simulink model "uavModelModifiedOld"  (R2019a)
settings: Solver=VariableStepAuto  StartTime=0.0  StopTime=50  RelTol=1e-3
undefined symbols (not defined in the file or in its folder): Motor
libraries: simulink x8
(part 1 of 2)
settings Model: Creator=tdarrah  LastModifiedBy=tdarrah
settings DataIOCC: ReturnWorkspaceOutputs=off
settings DebuggingCC: ArithmeticOperatorsInVariantConditions=warning
settings SFSimCC: SimUseLocalCustomCode=off
settings RTWCC: RTWUseLocalCustomCode=off
settings CodeAppCC: StateflowObjectComments=on

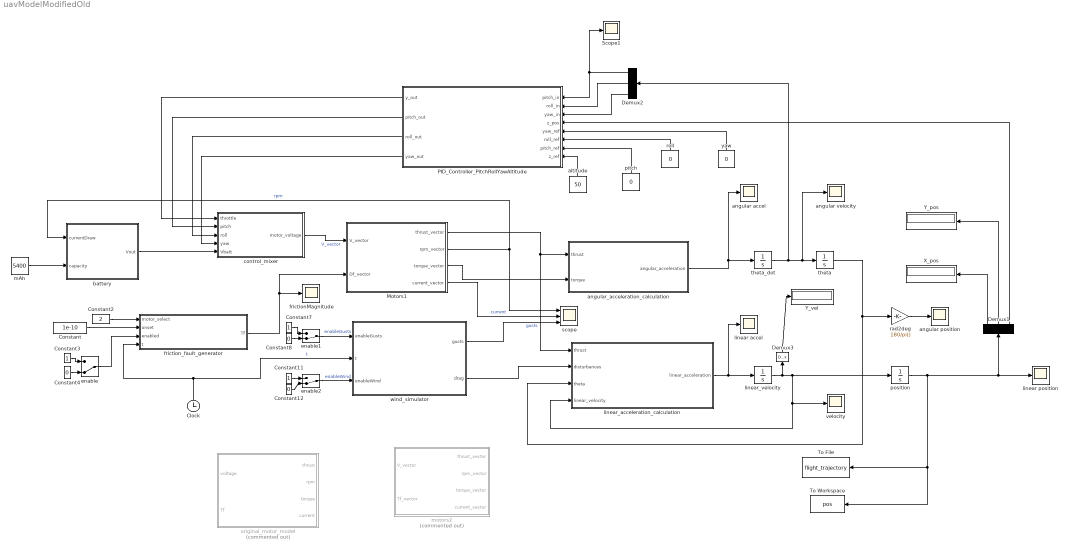
== system uavModelModifiedOld ==
  Clock : Clock
  Constant : Constant  Value=1e-10
  Constant11 : Constant
  Constant12 : Constant  Value=0
  Constant2 : Constant  Value=2
  Constant3 : Constant
  Constant4 : Constant  Value=0
  Constant7 : Constant
  Constant8 : Constant  Value=0
  Demux1 : Demux  Outputs=3
  Demux2 : Demux  Outputs=3
  Demux3 : Demux  Outputs=3
  Motors1 : Subsystem
  PID_Controller_PitchRollYawAltitude : Subsystem
  Scope1 : Scope
  To File : ToFile  Filename=flight_trajectory  MatrixName=pos  SampleTime=.1
  To Workspace : ToWorkspace  VariableName=pos  SampleTime=-1
      settings: Save2DSignal=2-D array (concatenate along first dimension)
  X_pos : Display
  Y_pos : Display
  Y_vel : Display
  altitude : Constant  Value=50
  angular accel : Scope
  angular position : Scope
  angular velocity : Scope
  angular_acceleration_calculation : MATLAB Function  TreatAsAtomicUnit=on
  battery : Subsystem
  control_mixer : MATLAB Function  TreatAsAtomicUnit=on
  enable : ManualSwitch  CurrentSetting=0
  enable1 : ManualSwitch  CurrentSetting=0
  enable2 : ManualSwitch  CurrentSetting=0
  frictionMagnitude : Scope
  friction_fault_generator : MATLAB Function  TreatAsAtomicUnit=on
  linear accel : Scope
  linear position : Scope
  linear_acceleration_calculation : MATLAB Function  TreatAsAtomicUnit=on
  linear_velocity : Integrator
  mAh : Constant  Value=5400
  motors2 : Subsystem  Commented=on
  original_motor_model : MATLAB Function  Commented=on  TreatAsAtomicUnit=on
  pitch : Constant  Value=0
  "position " : Integrator
  rad2deg : Gain  Gain=180/pi()
  roll : Constant  Value=0
  scope : Scope  NumInputPorts=3
  theta : Integrator
  theta_dot : Integrator
  velocity : Scope
  wind_simulator : Subsystem
  yaw : Constant  Value=0
  wires:
  Motors1/1(thrust_vector) -> linear_acceleration_calculation/1(thrust), angular_acceleration_calculation/1(thrust)
  Motors1/3(torque_vector) -> angular_acceleration_calculation/2(torque)
  angular_acceleration_calculation/1(angular_acceleration) -> angular accel/1, theta_dot/1
  theta_dot/1 -> Demux2/1, angular velocity/1, theta/1
  linear_acceleration_calculation/1(linear_acceleration) -> linear accel/1, linear_velocity/1
  linear_velocity/1 -> "position "/1, linear_acceleration_calculation/4(linear_velocity), velocity/1, Demux3/1
  rad2deg/1 -> angular position/1
  theta/1 -> rad2deg/1, linear_acceleration_calculation/3(theta)
  control_mixer/1(motor_voltage) -> Motors1/1(V_vector)  "V_vector"
  Motors1/4(current_vector) -> scope/2  "current"
  battery/1(Vout) -> control_mixer/5(Vbatt)
  Demux2/1 -> PID_Controller_PitchRollYawAltitude/1(pitch_in), Scope1/1
  Demux2/2 -> PID_Controller_PitchRollYawAltitude/2(roll_in)
  Demux2/3 -> PID_Controller_PitchRollYawAltitude/3(yaw_in)
  Demux1/3 -> PID_Controller_PitchRollYawAltitude/4(z_pos)
  PID_Controller_PitchRollYawAltitude/1(y_out) -> control_mixer/1(throttle)
  PID_Controller_PitchRollYawAltitude/2(pitch_out) -> control_mixer/2(pitch)
  PID_Controller_PitchRollYawAltitude/3(roll_out) -> control_mixer/3(roll)
  PID_Controller_PitchRollYawAltitude/4(yaw_out) -> control_mixer/4(yaw)
  altitude/1 -> PID_Controller_PitchRollYawAltitude/8(z_ref)
  roll/1 -> PID_Controller_PitchRollYawAltitude/6(roll_ref)
  yaw/1 -> PID_Controller_PitchRollYawAltitude/5(yaw_ref)
  Clock/1 -> wind_simulator/2(t), friction_fault_generator/4(t)  "t"
  friction_fault_generator/1(Tf) -> frictionMagnitude/1, Motors1/2(Df_vector)
  Constant2/1 -> friction_fault_generator/1(motor_select)
  Constant3/1 -> enable/1
  enable/1 -> friction_fault_generator/3(enabled)
  Constant4/1 -> enable/2
  Motors1/2(rpm_vector) -> battery/1(currentDraw), scope/1  "rpm"
  "position "/1 -> linear position/1, Demux1/1, To File/1, To Workspace/1
  Constant/1 -> friction_fault_generator/2(onset)
  mAh/1 -> battery/2(capacity)
  wind_simulator/1(gusts) -> scope/3  "gusts"
  wind_simulator/2(drag) -> linear_acceleration_calculation/2(disturbances)
  Demux1/1 -> X_pos/1
  Demux1/2 -> Y_pos/1
  Constant7/1 -> enable1/1
  Constant8/1 -> enable1/2
  enable1/1 -> wind_simulator/1(enableGusts)  "enableGusts"
  Constant11/1 -> enable2/1
  enable2/1 -> wind_simulator/3(enableWind)  "enableWind"
  Constant12/1 -> enable2/2
  Demux3/2 -> Y_vel/1
  pitch/1 -> PID_Controller_PitchRollYawAltitude/7(pitch_ref)

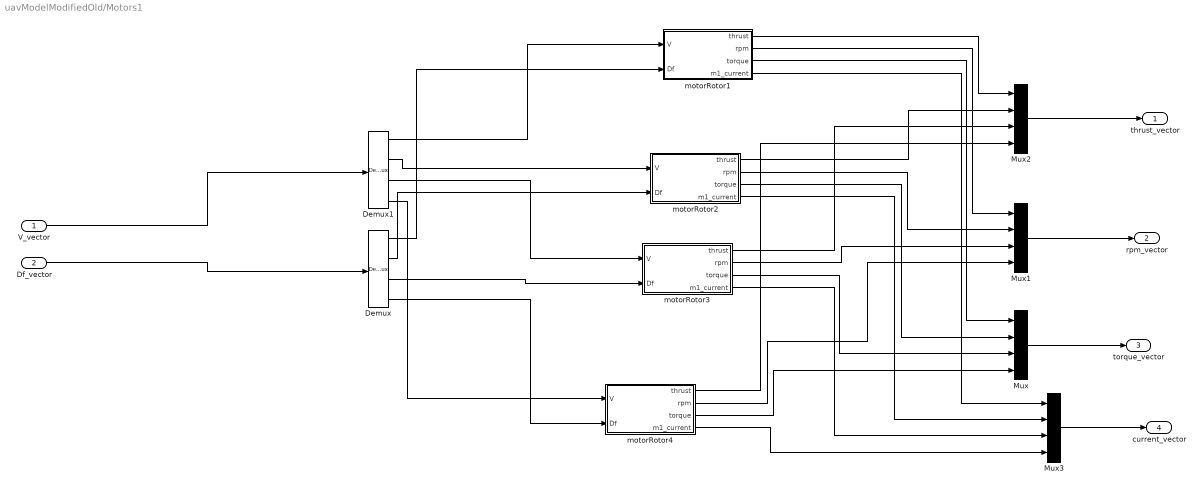
== system uavModelModifiedOld/Motors1 ==
  V_vector : Inport
  Df_vector : Inport  Port=2
  Demux : Demux
  Demux1 : Demux
  Mux{,1..3} (4 alike) : Mux
  motorRotor1 : Subsystem
  motorRotor2 : Subsystem
  motorRotor3 : Subsystem
  motorRotor4 : Subsystem
  thrust_vector : Outport
  rpm_vector : Outport  Port=2
  torque_vector : Outport  Port=3
  current_vector : Outport  Port=4
  wires:
  motorRotor4/3(torque) -> Mux/4
  motorRotor1/2(rpm) -> Mux1/1
  Mux1/1 -> rpm_vector/1
  Demux1/3 -> motorRotor3/1(V)
  V_vector/1 -> Demux1/1
  motorRotor1/1(thrust) -> Mux2/1
  motorRotor4/1(thrust) -> Mux2/4
  motorRotor3/2(rpm) -> Mux1/3
  motorRotor2/2(rpm) -> Mux1/2
  motorRotor2/3(torque) -> Mux/2
  Mux2/1 -> thrust_vector/1
  motorRotor1/3(torque) -> Mux/1
  motorRotor3/3(torque) -> Mux/3
  motorRotor4/2(rpm) -> Mux1/4
  motorRotor2/1(thrust) -> Mux2/2
  motorRotor3/1(thrust) -> Mux2/3
  Demux1/1 -> motorRotor1/1(V)
  Demux/2 -> motorRotor2/2(Df)
  Demux/3 -> motorRotor3/2(Df)
  Demux/1 -> motorRotor1/2(Df)
  Df_vector/1 -> Demux/1
  Demux1/4 -> motorRotor4/1(V)
  Mux/1 -> torque_vector/1
  Demux1/2 -> motorRotor2/1(V)
  Demux/4 -> motorRotor4/2(Df)
  motorRotor1/4(m1_current) -> Mux3/1
  Mux3/1 -> current_vector/1
  motorRotor2/4(m1_current) -> Mux3/2
  motorRotor3/4(m1_current) -> Mux3/3
  motorRotor4/4(m1_current) -> Mux3/4

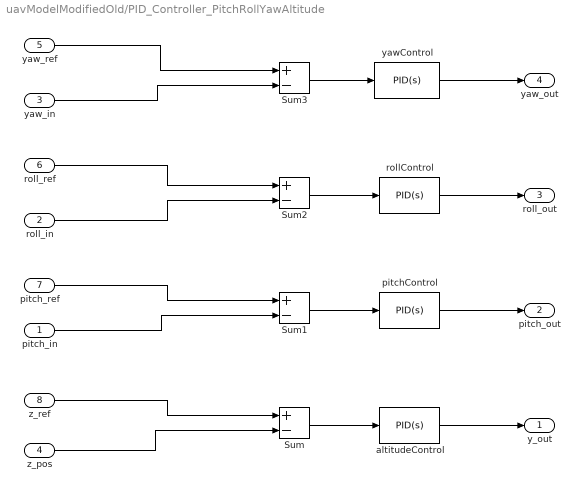
== system uavModelModifiedOld/PID_Controller_PitchRollYawAltitude ==
  pitch_in : Inport
  roll_in : Inport  Port=2
  yaw_in : Inport  Port=3
  z_pos : Inport  Port=4
  yaw_ref : Inport  Port=5
  roll_ref : Inport  Port=6
  pitch_ref : Inport  Port=7
  z_ref : Inport  Port=8
  Sum{,1..3} (4 alike) : Sum  Inputs=+-
  altitudeControl : simulink/Continuous/PID Controller  Controller=PID  Form=Parallel  TimeDomain=Continuous-time  SampleTime=-1  IntegratorMethod=Forward Euler  FilterMethod=Forward Euler  ControllerParametersSource=internal  P=9.031  I=1  D=10  UseFilter=on  N=100  TunerSelectOption=Transfer Function Based (PID Tuner App)  InitialConditionSource=internal  InitialConditionForIntegrator=0  InitialConditionForFilter=0  DifferentiatorICPrevScaledInput=0  ExternalReset=none  TrackingMode=off  Kt=1  LimitOutput=on  UpperSaturationLimit=100  LowerSaturationLimit=0  LinearizeAsGain=on  AntiWindupMode=clamping  Kb=1  POutMin=[]  POutMax=[]  IOutMin=[]  IOutMax=[]  DOutMin=[]  DOutMax=[]  NOutMin=[]  NOutMax=[]  SumOutMin=[]  SumOutMax=[]  SaturationOutMin=[]  SaturationOutMax=[]  PParamMin=[]  PParamMax=[]  IParamMin=[]  IParamMax=[]  DParamMin=[]  DParamMax=[]  NParamMin=[]  NParamMax=[]  KbParamMin=[]  KbParamMax=[]  KtParamMin=[]  KtParamMax=[]  KbOutMin=[]  KbOutMax=[]  KtOutMin=[]  KtOutMax=[]  IntegratorOutMin=[]  IntegratorOutMax=[]  FilterOutMin=[]  FilterOutMax=[]  SumI1OutMin=[]  SumI1OutMax=[]  SumI2OutMin=[]  SumI2OutMax=[]  SumI3OutMin=[]  SumI3OutMax=[]  SumI4OutMin=[]  SumI4OutMax=[]  SumDOutMin=[]  SumDOutMax=[]  DifferentiatorOutMin=[]  DifferentiatorOutMax=[]  FilterDiffOutCoefMin=[]  FilterDiffOutCoefMax=[]  ReciprocalOutMin=[]  ReciprocalOutMax=[]  SumDenOutMin=[]  SumDenOutMax=[]  SumNumOutMin=[]  SumNumOutMax=[]  DivideOutMin=[]  DivideOutMax=[]  IntegratorContinuousStateAttributes=''  IntegratorStateMustResolveToSignalObject=off  IntegratorRTWStateStorageClass=Auto  FilterContinuousStateAttributes=''  FilterStateMustResolveToSignalObject=off  FilterRTWStateStorageClass=Auto  ParallelPVariant=InternalParameters  IdealPVariant=Disabled  IVariant=InternalParameters  DVariant=InternalParameters  IntegratorVariant=Continuous  SatVariant=Enabled  AWVariant=ContClampingParallel  PCopyVariant=Disabled  TRVariant=Disabled  FdbkBlocksVariant=Forward  IdealPFdbkVariant=Disabled  SatFdbkVariant=Disabled  DerivativeFilterVariant=ContFilter  NVariant=InternalParameters  NCopyVariant=Disabled  FilterICVariant=InternalICsFilter  IntegratorICVariant=InternalICs  ExternalResetVariant=Disabled  TRSumVariant=Passthrough  SumFdbkVariant=Disabled  SumVariant=Sum_PID
  pitchControl : simulink/Continuous/PID Controller  Controller=PID  Form=Parallel  TimeDomain=Continuous-time  SampleTime=-1  IntegratorMethod=Forward Euler  FilterMethod=Forward Euler  ControllerParametersSource=internal  P=15  I=5  D=0  UseFilter=on  N=100  TunerSelectOption=Transfer Function Based (PID Tuner App)  InitialConditionSource=internal  InitialConditionForIntegrator=0  InitialConditionForFilter=0  DifferentiatorICPrevScaledInput=0  ExternalReset=none  TrackingMode=off  Kt=1  LimitOutput=on  UpperSaturationLimit=100  LowerSaturationLimit=0  LinearizeAsGain=on  AntiWindupMode=clamping  Kb=1  POutMin=[]  POutMax=[]  IOutMin=[]  IOutMax=[]  DOutMin=[]  DOutMax=[]  NOutMin=[]  NOutMax=[]  SumOutMin=[]  SumOutMax=[]  SaturationOutMin=[]  SaturationOutMax=[]  PParamMin=[]  PParamMax=[]  IParamMin=[]  IParamMax=[]  DParamMin=[]  DParamMax=[]  NParamMin=[]  NParamMax=[]  KbParamMin=[]  KbParamMax=[]  KtParamMin=[]  KtParamMax=[]  KbOutMin=[]  KbOutMax=[]  KtOutMin=[]  KtOutMax=[]  IntegratorOutMin=[]  IntegratorOutMax=[]  FilterOutMin=[]  FilterOutMax=[]  SumI1OutMin=[]  SumI1OutMax=[]  SumI2OutMin=[]  SumI2OutMax=[]  SumI3OutMin=[]  SumI3OutMax=[]  SumI4OutMin=[]  SumI4OutMax=[]  SumDOutMin=[]  SumDOutMax=[]  DifferentiatorOutMin=[]  DifferentiatorOutMax=[]  FilterDiffOutCoefMin=[]  FilterDiffOutCoefMax=[]  ReciprocalOutMin=[]  ReciprocalOutMax=[]  SumDenOutMin=[]  SumDenOutMax=[]  SumNumOutMin=[]  SumNumOutMax=[]  DivideOutMin=[]  DivideOutMax=[]  IntegratorContinuousStateAttributes=''  IntegratorStateMustResolveToSignalObject=off  IntegratorRTWStateStorageClass=Auto  FilterContinuousStateAttributes=''  FilterStateMustResolveToSignalObject=off  FilterRTWStateStorageClass=Auto  ParallelPVariant=InternalParameters  IdealPVariant=Disabled  IVariant=InternalParameters  DVariant=InternalParameters  IntegratorVariant=Continuous  SatVariant=Enabled  AWVariant=ContClampingParallel  PCopyVariant=Disabled  TRVariant=Disabled  FdbkBlocksVariant=Forward  IdealPFdbkVariant=Disabled  SatFdbkVariant=Disabled  DerivativeFilterVariant=ContFilter  NVariant=InternalParameters  NCopyVariant=Disabled  FilterICVariant=InternalICsFilter  IntegratorICVariant=InternalICs  ExternalResetVariant=Disabled  TRSumVariant=Passthrough  SumFdbkVariant=Disabled  SumVariant=Sum_PID
  rollControl : simulink/Continuous/PID Controller  Controller=PID  Form=Parallel  TimeDomain=Continuous-time  SampleTime=-1  IntegratorMethod=Forward Euler  FilterMethod=Forward Euler  ControllerParametersSource=internal  P=15  I=5  D=0  UseFilter=on  N=100  TunerSelectOption=Transfer Function Based (PID Tuner App)  InitialConditionSource=internal  InitialConditionForIntegrator=0  InitialConditionForFilter=0  DifferentiatorICPrevScaledInput=0  ExternalReset=none  TrackingMode=off  Kt=1  LimitOutput=on  UpperSaturationLimit=100  LowerSaturationLimit=0  LinearizeAsGain=on  AntiWindupMode=clamping  Kb=1  POutMin=[]  POutMax=[]  IOutMin=[]  IOutMax=[]  DOutMin=[]  DOutMax=[]  NOutMin=[]  NOutMax=[]  SumOutMin=[]  SumOutMax=[]  SaturationOutMin=[]  SaturationOutMax=[]  PParamMin=[]  PParamMax=[]  IParamMin=[]  IParamMax=[]  DParamMin=[]  DParamMax=[]  NParamMin=[]  NParamMax=[]  KbParamMin=[]  KbParamMax=[]  KtParamMin=[]  KtParamMax=[]  KbOutMin=[]  KbOutMax=[]  KtOutMin=[]  KtOutMax=[]  IntegratorOutMin=[]  IntegratorOutMax=[]  FilterOutMin=[]  FilterOutMax=[]  SumI1OutMin=[]  SumI1OutMax=[]  SumI2OutMin=[]  SumI2OutMax=[]  SumI3OutMin=[]  SumI3OutMax=[]  SumI4OutMin=[]  SumI4OutMax=[]  SumDOutMin=[]  SumDOutMax=[]  DifferentiatorOutMin=[]  DifferentiatorOutMax=[]  FilterDiffOutCoefMin=[]  FilterDiffOutCoefMax=[]  ReciprocalOutMin=[]  ReciprocalOutMax=[]  SumDenOutMin=[]  SumDenOutMax=[]  SumNumOutMin=[]  SumNumOutMax=[]  DivideOutMin=[]  DivideOutMax=[]  IntegratorContinuousStateAttributes=''  IntegratorStateMustResolveToSignalObject=off  IntegratorRTWStateStorageClass=Auto  FilterContinuousStateAttributes=''  FilterStateMustResolveToSignalObject=off  FilterRTWStateStorageClass=Auto  ParallelPVariant=InternalParameters  IdealPVariant=Disabled  IVariant=InternalParameters  DVariant=InternalParameters  IntegratorVariant=Continuous  SatVariant=Enabled  AWVariant=ContClampingParallel  PCopyVariant=Disabled  TRVariant=Disabled  FdbkBlocksVariant=Forward  IdealPFdbkVariant=Disabled  SatFdbkVariant=Disabled  DerivativeFilterVariant=ContFilter  NVariant=InternalParameters  NCopyVariant=Disabled  FilterICVariant=InternalICsFilter  IntegratorICVariant=InternalICs  ExternalResetVariant=Disabled  TRSumVariant=Passthrough  SumFdbkVariant=Disabled  SumVariant=Sum_PID
  yawControl : simulink/Continuous/PID Controller  Controller=PID  Form=Parallel  TimeDomain=Continuous-time  SampleTime=-1  IntegratorMethod=Forward Euler  FilterMethod=Forward Euler  ControllerParametersSource=internal  P=15  I=5  D=0  UseFilter=on  N=100  TunerSelectOption=Transfer Function Based (PID Tuner App)  InitialConditionSource=internal  InitialConditionForIntegrator=0  InitialConditionForFilter=0  DifferentiatorICPrevScaledInput=0  ExternalReset=none  TrackingMode=off  Kt=1  LimitOutput=on  UpperSaturationLimit=100  LowerSaturationLimit=0  LinearizeAsGain=on  AntiWindupMode=clamping  Kb=1  POutMin=[]  POutMax=[]  IOutMin=[]  IOutMax=[]  DOutMin=[]  DOutMax=[]  NOutMin=[]  NOutMax=[]  SumOutMin=[]  SumOutMax=[]  SaturationOutMin=[]  SaturationOutMax=[]  PParamMin=[]  PParamMax=[]  IParamMin=[]  IParamMax=[]  DParamMin=[]  DParamMax=[]  NParamMin=[]  NParamMax=[]  KbParamMin=[]  KbParamMax=[]  KtParamMin=[]  KtParamMax=[]  KbOutMin=[]  KbOutMax=[]  KtOutMin=[]  KtOutMax=[]  IntegratorOutMin=[]  IntegratorOutMax=[]  FilterOutMin=[]  FilterOutMax=[]  SumI1OutMin=[]  SumI1OutMax=[]  SumI2OutMin=[]  SumI2OutMax=[]  SumI3OutMin=[]  SumI3OutMax=[]  SumI4OutMin=[]  SumI4OutMax=[]  SumDOutMin=[]  SumDOutMax=[]  DifferentiatorOutMin=[]  DifferentiatorOutMax=[]  FilterDiffOutCoefMin=[]  FilterDiffOutCoefMax=[]  ReciprocalOutMin=[]  ReciprocalOutMax=[]  SumDenOutMin=[]  SumDenOutMax=[]  SumNumOutMin=[]  SumNumOutMax=[]  DivideOutMin=[]  DivideOutMax=[]  IntegratorContinuousStateAttributes=''  IntegratorStateMustResolveToSignalObject=off  IntegratorRTWStateStorageClass=Auto  FilterContinuousStateAttributes=''  FilterStateMustResolveToSignalObject=off  FilterRTWStateStorageClass=Auto  ParallelPVariant=InternalParameters  IdealPVariant=Disabled  IVariant=InternalParameters  DVariant=InternalParameters  IntegratorVariant=Continuous  SatVariant=Enabled  AWVariant=ContClampingParallel  PCopyVariant=Disabled  TRVariant=Disabled  FdbkBlocksVariant=Forward  IdealPFdbkVariant=Disabled  SatFdbkVariant=Disabled  DerivativeFilterVariant=ContFilter  NVariant=InternalParameters  NCopyVariant=Disabled  FilterICVariant=InternalICsFilter  IntegratorICVariant=InternalICs  ExternalResetVariant=Disabled  TRSumVariant=Passthrough  SumFdbkVariant=Disabled  SumVariant=Sum_PID
  y_out : Outport
  pitch_out : Outport  Port=2
  roll_out : Outport  Port=3
  yaw_out : Outport  Port=4
  wires:
  yawControl/1 -> yaw_out/1
  Sum3/1 -> yawControl/1
  roll_ref/1 -> Sum2/1
  pitch_in/1 -> Sum1/2
  roll_in/1 -> Sum2/2
  yaw_in/1 -> Sum3/2
  rollControl/1 -> roll_out/1
  pitch_ref/1 -> Sum1/1
  Sum1/1 -> pitchControl/1
  z_pos/1 -> Sum/2
  Sum/1 -> altitudeControl/1
  yaw_ref/1 -> Sum3/1
  Sum2/1 -> rollControl/1
  pitchControl/1 -> pitch_out/1
  altitudeControl/1 -> y_out/1
  z_ref/1 -> Sum/1

== system uavModelModifiedOld/battery ==
  currentDraw : Inport
  capacity : Inport  Port=2
  Constant1 : Constant  Value=11.4
  Vout : Outport
  wires:
  Constant1/1 -> Vout/1

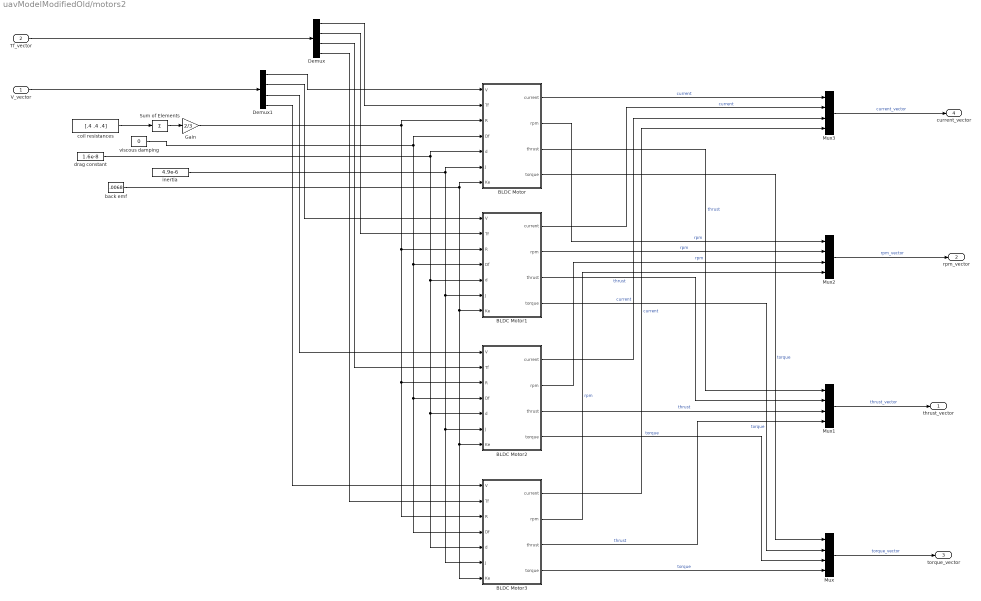
== system uavModelModifiedOld/motors2 ==
  V_vector : Inport
  Tf_vector : Inport  Port=2
  BLDC Motor : Subsystem
  BLDC Motor1 : Subsystem
  BLDC Motor2 : Subsystem
  BLDC Motor3 : Subsystem
  Demux : Demux
  Demux1 : Demux
  Gain : Gain  Gain=2/3
  Mux{,1..3} (4 alike) : Mux
  Sum of Elements : Sum  Inputs=+
  back emf : Constant  Value=.0068
  coil resistances : Constant  Value=[.4 .4 .4]
  drag constant : Constant  Value=1.6e-8
  inertia : Constant  Value=4.9e-6
  viscous damping : Constant  Value=0
  thrust_vector : Outport
  rpm_vector : Outport  Port=2
  torque_vector : Outport  Port=3
  current_vector : Outport  Port=4
  wires:
  BLDC Motor/2(rpm) -> Mux2/1  "rpm"
  Demux1/3 -> BLDC Motor2/1(V)
  BLDC Motor/1(current) -> Mux3/1  "current"
  BLDC Motor3/3(thrust) -> Mux1/4  "thrust"
  V_vector/1 -> Demux1/1
  Demux1/2 -> BLDC Motor1/1(V)
  BLDC Motor/3(thrust) -> Mux1/1  "thrust"
  Demux1/4 -> BLDC Motor3/1(V)
  BLDC Motor/4(torque) -> Mux/1  "torque"
  Mux2/1 -> rpm_vector/1  "rpm_vector"
  back emf/1 -> BLDC Motor/7(Ke), BLDC Motor3/7(Ke), BLDC Motor2/7(Ke), BLDC Motor1/7(Ke)
  Demux/2 -> BLDC Motor1/2(Tf)
  BLDC Motor2/3(thrust) -> Mux1/3  "thrust"
  Gain/1 -> BLDC Motor/3(R), BLDC Motor3/3(R), BLDC Motor2/3(R), BLDC Motor1/3(R)
  BLDC Motor1/1(current) -> Mux3/2  "current"
  inertia/1 -> BLDC Motor/6(J), BLDC Motor3/6(J), BLDC Motor2/6(J), BLDC Motor1/6(J)
  Tf_vector/1 -> Demux/1
  Demux/1 -> BLDC Motor/2(Tf)
  viscous damping/1 -> BLDC Motor/4(Df), BLDC Motor3/4(Df), BLDC Motor2/4(Df), BLDC Motor1/4(Df)
  BLDC Motor2/1(current) -> Mux3/3  "current"
  Mux3/1 -> current_vector/1  "current_vector"
  BLDC Motor1/3(thrust) -> Mux1/2  "thrust"
  Mux1/1 -> thrust_vector/1  "thrust_vector"
  BLDC Motor2/2(rpm) -> Mux2/3  "rpm"
  Demux/4 -> BLDC Motor3/2(Tf)
  BLDC Motor2/4(torque) -> Mux/3  "torque"
  Sum of Elements/1 -> Gain/1
  BLDC Motor1/2(rpm) -> Mux2/2  "rpm"
  Mux/1 -> torque_vector/1  "torque_vector"
  Demux/3 -> BLDC Motor2/2(Tf)
  BLDC Motor1/4(torque) -> Mux/2  "torque"
  BLDC Motor3/1(current) -> Mux3/4  "current"
  Demux1/1 -> BLDC Motor/1(V)
  BLDC Motor3/4(torque) -> Mux/4  "torque"
  BLDC Motor3/2(rpm) -> Mux2/4  "rpm"
  drag constant/1 -> BLDC Motor/5(d), BLDC Motor3/5(d), BLDC Motor2/5(d), BLDC Motor1/5(d)
  coil resistances/1 -> Sum of Elements/1

== system uavModelModifiedOld/wind_simulator ==
  enableGusts : Inport
  t : Inport  Port=2
  enableWind : Inport  Port=3
  Constant10 : Constant
  Constant5 : Constant  Value=5
  Constant6 : Constant  Value=4
  Constant9 : Constant
  wind_and_gust : Subsystem
  gusts : Outport
  drag : Outport  Port=2
  wires:
  enableGusts/1 -> wind_and_gust/1(enableGusts)  "enableGusts"
  wind_and_gust/2(drag) -> drag/1  "drag"
  Constant6/1 -> wind_and_gust/3(amplitude)  "amplitude"
  Constant10/1 -> wind_and_gust/6(speed)  "speed"
  Constant9/1 -> wind_and_gust/5(windDirection)  "windDirection"
  wind_and_gust/1(gusts) -> gusts/1  "gusts"
  enableWind/1 -> wind_and_gust/7(enableWind)  "enableWind"
  t/1 -> wind_and_gust/4(t)
  Constant5/1 -> wind_and_gust/2(period)  "period"

== system uavModelModifiedOld/Motors1/motorRotor1 ==
  V : Inport
  Df : Inport  Port=2
  Convert rad/s to rmp : Gain  Gain=60/(2*pi)
  Electrical part : Subsystem
  Mechanical part : Subsystem
  thrust : Outport
  rpm : Outport  Port=2
  torque : Outport  Port=3
  m1_current : Outport  Port=4
  wires:
  Convert rad/s to rmp/1 -> rpm/1
  V/1 -> Electrical part/1(ESC voltage)
  Mechanical part/2(Thrust) -> thrust/1
  Electrical part/1(Electrical Torque) -> Mechanical part/2(Electrical Torque)
  Mechanical part/3(Torque) -> torque/1
  Mechanical part/1(w angular speed) -> Electrical part/2(w angular speed), Convert rad/s to rmp/1
  Df/1 -> Mechanical part/1(dynamicFriction)
  Electrical part/2(current) -> m1_current/1

== system uavModelModifiedOld/Motors1/motorRotor2 ==
  V : Inport
  Df : Inport  Port=2
  Convert rad/s to rmp : Gain  Gain=60/(2*pi)
  Electrical part : Subsystem
  Mechanical part : Subsystem
  thrust : Outport
  rpm : Outport  Port=2
  torque : Outport  Port=3
  m1_current : Outport  Port=4
  wires:
  Convert rad/s to rmp/1 -> rpm/1
  V/1 -> Electrical part/1(ESC voltage)
  Mechanical part/2(Thrust) -> thrust/1
  Electrical part/1(Electrical Torque) -> Mechanical part/2(Electrical Torque)
  Mechanical part/3(Torque) -> torque/1
  Mechanical part/1(w angular speed) -> Electrical part/2(w angular speed), Convert rad/s to rmp/1
  Df/1 -> Mechanical part/1(dynamicFriction)
  Electrical part/2(current) -> m1_current/1

== system uavModelModifiedOld/Motors1/motorRotor3 ==
  V : Inport
  Df : Inport  Port=2
  Convert rad/s to rmp : Gain  Gain=60/(2*pi)
  Electrical part : Subsystem
  Mechanical part : Subsystem
  thrust : Outport
  rpm : Outport  Port=2
  torque : Outport  Port=3
  m1_current : Outport  Port=4
  wires:
  Convert rad/s to rmp/1 -> rpm/1
  V/1 -> Electrical part/1(ESC voltage)
  Mechanical part/2(Thrust) -> thrust/1
  Electrical part/1(Electrical Torque) -> Mechanical part/2(Electrical Torque)
  Mechanical part/3(Torque) -> torque/1
  Mechanical part/1(w angular speed) -> Electrical part/2(w angular speed), Convert rad/s to rmp/1
  Df/1 -> Mechanical part/1(dynamicFriction)
  Electrical part/2(current) -> m1_current/1

== system uavModelModifiedOld/Motors1/motorRotor4 ==
  V : Inport
  Df : Inport  Port=2
  Convert rad/s to rmp : Gain  Gain=60/(2*pi)
  Electrical part : Subsystem
  Mechanical part : Subsystem
  thrust : Outport
  rpm : Outport  Port=2
  torque : Outport  Port=3
  m1_current : Outport  Port=4
  wires:
  Convert rad/s to rmp/1 -> rpm/1
  V/1 -> Electrical part/1(ESC voltage)
  Mechanical part/2(Thrust) -> thrust/1
  Electrical part/1(Electrical Torque) -> Mechanical part/2(Electrical Torque)
  Mechanical part/3(Torque) -> torque/1
  Mechanical part/1(w angular speed) -> Electrical part/2(w angular speed), Convert rad/s to rmp/1
  Df/1 -> Mechanical part/1(dynamicFriction)
  Electrical part/2(current) -> m1_current/1

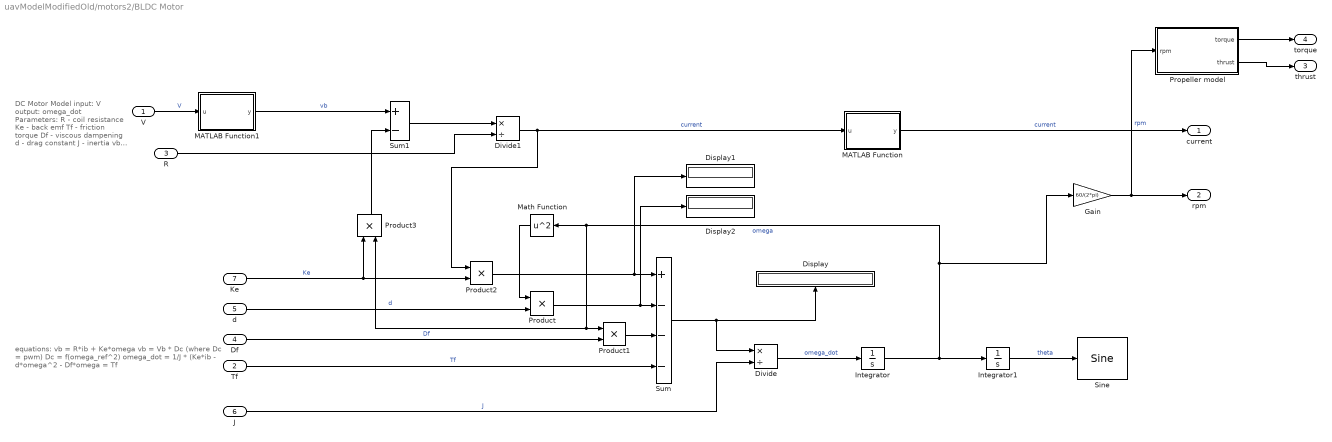
== system uavModelModifiedOld/motors2/BLDC Motor ==
  note: DC Motor Model
      |
      | input:
      | V
      |
      | output:
      | omega_dot
      |
      | Parameters:
      | R   - coil resistance
      | Ke - back emf
      | Tf  - friction torque
      | Df  - viscous dampening
      | d   - drag constant
      | J   - inertia
      |
      |
      | vb - average battery voltage
      | ib  - average battery current
  note: equations:
      |
      | vb = R*ib + Ke*omega
      | vb = Vb * Dc  (where Dc = pwm)
      | Dc = f(omega_ref^2)
      |
      | omega_dot = 1/J * (Ke*ib - d*omega^2 - Df*omega = Tf
  V : Inport
  Tf : Inport  Port=2
  R : Inport  Port=3
  Df : Inport  Port=4
  d : Inport  Port=5
  J : Inport  Port=6
  Ke : Inport  Port=7
  Display : Display
  Display1 : Display
  Display2 : Display
  Divide : Product  Inputs=*/
  Divide1 : Product  Inputs=*/
  Gain : Gain  Gain=60/(2*pi)
  Integrator : Integrator
  Integrator1 : Integrator
  MATLAB Function : MATLAB Function  TreatAsAtomicUnit=on
  MATLAB Function1 : MATLAB Function  TreatAsAtomicUnit=on
  Math Function : Math  Operator=square  SaturateOnIntegerOverflow=on
  Product{,1..3} (4 alike) : Product
  "Propeller model " : MATLAB Function  TreatAsAtomicUnit=on
  Sine : simulink/Lookup Tables/Sine  Formula=sin(2*pi*u)  NumDataPoints=180  OutputWordLength=16  InternalRulePriority=Speed
      settings: SourceProductName=Simulink
  Sum : Sum  Inputs=+---
  Sum1 : Sum  Inputs=+-
  current : Outport
  rpm : Outport  Port=2
  thrust : Outport  Port=3
  torque : Outport  Port=4
  wires:
  Divide/1 -> Integrator/1  "omega_dot"
  Integrator/1 -> Gain/1, Math Function/1, Product1/1, Product3/2, Integrator1/1  "omega"
  Integrator1/1 -> Sine/1  "theta"
  Gain/1 -> "Propeller model "/1(rpm), rpm/1  "rpm"
  J/1 -> Divide/2  "J"
  d/1 -> Product/2  "d"
  Math Function/1 -> Product/1
  Df/1 -> Product1/2  "Df"
  Tf/1 -> Sum/4  "Tf"
  Ke/1 -> Product3/1, Product2/2  "Ke"
  Product2/1 -> Display1/1, Sum/1
  Divide1/1 -> Product2/1, MATLAB Function/1(u)  "current"
  V/1 -> MATLAB Function1/1(u)  "V"
  Product3/1 -> Sum1/2
  MATLAB Function/1(y) -> current/1  "current"
  MATLAB Function1/1(y) -> Sum1/1  "vb"
  Sum1/1 -> Divide1/1
  R/1 -> Divide1/2
  "Propeller model "/2(thrust) -> thrust/1
  "Propeller model "/1(torque) -> torque/1
  Product1/1 -> Sum/3
  Product/1 -> Display2/1, Sum/2
  Sum/1 -> Display/1, Divide/1

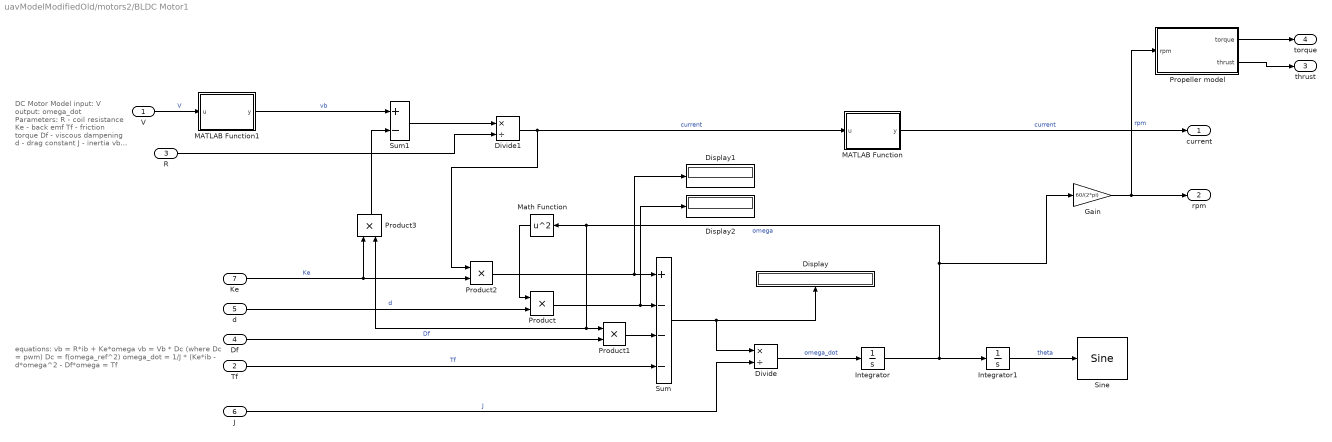
== system uavModelModifiedOld/motors2/BLDC Motor1 ==
  note: DC Motor Model
      |
      | input:
      | V
      |
      | output:
      | omega_dot
      |
      | Parameters:
      | R   - coil resistance
      | Ke - back emf
      | Tf  - friction torque
      | Df  - viscous dampening
      | d   - drag constant
      | J   - inertia
      |
      |
      | vb - average battery voltage
      | ib  - average battery current
  note: equations:
      |
      | vb = R*ib + Ke*omega
      | vb = Vb * Dc  (where Dc = pwm)
      | Dc = f(omega_ref^2)
      |
      | omega_dot = 1/J * (Ke*ib - d*omega^2 - Df*omega = Tf
  V : Inport
  Tf : Inport  Port=2
  R : Inport  Port=3
  Df : Inport  Port=4
  d : Inport  Port=5
  J : Inport  Port=6
  Ke : Inport  Port=7
  Display : Display
  Display1 : Display
  Display2 : Display
  Divide : Product  Inputs=*/
  Divide1 : Product  Inputs=*/
  Gain : Gain  Gain=60/(2*pi)
  Integrator : Integrator
  Integrator1 : Integrator
  MATLAB Function : MATLAB Function  TreatAsAtomicUnit=on
  MATLAB Function1 : MATLAB Function  TreatAsAtomicUnit=on
  Math Function : Math  Operator=square  SaturateOnIntegerOverflow=on
  Product{,1..3} (4 alike) : Product
  "Propeller model " : MATLAB Function  TreatAsAtomicUnit=on
  Sine : simulink/Lookup Tables/Sine  Formula=sin(2*pi*u)  NumDataPoints=180  OutputWordLength=16  InternalRulePriority=Speed
      settings: SourceProductName=Simulink
  Sum : Sum  Inputs=+---
  Sum1 : Sum  Inputs=+-
  current : Outport
  rpm : Outport  Port=2
  thrust : Outport  Port=3
  torque : Outport  Port=4
  wires:
  Divide/1 -> Integrator/1  "omega_dot"
  Integrator/1 -> Gain/1, Math Function/1, Product1/1, Product3/2, Integrator1/1  "omega"
  Integrator1/1 -> Sine/1  "theta"
  Gain/1 -> "Propeller model "/1(rpm), rpm/1  "rpm"
  J/1 -> Divide/2  "J"
  d/1 -> Product/2  "d"
  Math Function/1 -> Product/1
  Df/1 -> Product1/2  "Df"
  Tf/1 -> Sum/4  "Tf"
  Ke/1 -> Product3/1, Product2/2  "Ke"
  Product2/1 -> Display1/1, Sum/1
  Divide1/1 -> Product2/1, MATLAB Function/1(u)  "current"
  V/1 -> MATLAB Function1/1(u)  "V"
  Product3/1 -> Sum1/2
  MATLAB Function/1(y) -> current/1  "current"
  MATLAB Function1/1(y) -> Sum1/1  "vb"
  Sum1/1 -> Divide1/1
  R/1 -> Divide1/2
  "Propeller model "/2(thrust) -> thrust/1
  "Propeller model "/1(torque) -> torque/1
  Product1/1 -> Sum/3
  Product/1 -> Display2/1, Sum/2
  Sum/1 -> Display/1, Divide/1

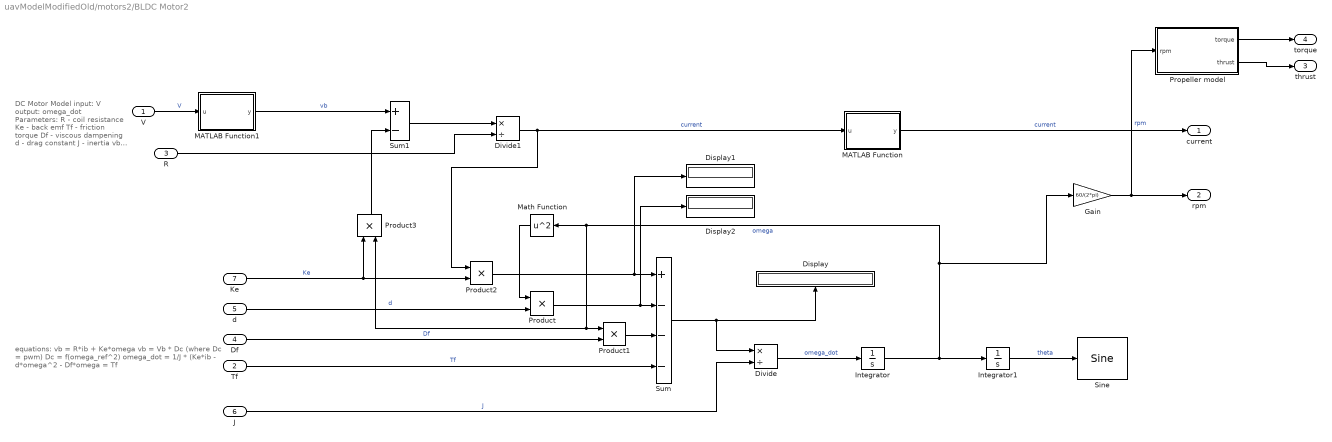
== system uavModelModifiedOld/motors2/BLDC Motor2 ==
  note: DC Motor Model
      |
      | input:
      | V
      |
      | output:
      | omega_dot
      |
      | Parameters:
      | R   - coil resistance
      | Ke - back emf
      | Tf  - friction torque
      | Df  - viscous dampening
      | d   - drag constant
      | J   - inertia
      |
      |
      | vb - average battery voltage
      | ib  - average battery current
  note: equations:
      |
      | vb = R*ib + Ke*omega
      | vb = Vb * Dc  (where Dc = pwm)
      | Dc = f(omega_ref^2)
      |
      | omega_dot = 1/J * (Ke*ib - d*omega^2 - Df*omega = Tf
  V : Inport
  Tf : Inport  Port=2
  R : Inport  Port=3
  Df : Inport  Port=4
  d : Inport  Port=5
  J : Inport  Port=6
  Ke : Inport  Port=7
  Display : Display
  Display1 : Display
  Display2 : Display
  Divide : Product  Inputs=*/
  Divide1 : Product  Inputs=*/
  Gain : Gain  Gain=60/(2*pi)
  Integrator : Integrator
  Integrator1 : Integrator
  MATLAB Function : MATLAB Function  TreatAsAtomicUnit=on
  MATLAB Function1 : MATLAB Function  TreatAsAtomicUnit=on
  Math Function : Math  Operator=square  SaturateOnIntegerOverflow=on
  Product{,1..3} (4 alike) : Product
  "Propeller model " : MATLAB Function  TreatAsAtomicUnit=on
  Sine : simulink/Lookup Tables/Sine  Formula=sin(2*pi*u)  NumDataPoints=180  OutputWordLength=16  InternalRulePriority=Speed
      settings: SourceProductName=Simulink
  Sum : Sum  Inputs=+---
  Sum1 : Sum  Inputs=+-
  current : Outport
  rpm : Outport  Port=2
  thrust : Outport  Port=3
  torque : Outport  Port=4
  wires:
  Divide/1 -> Integrator/1  "omega_dot"
  Integrator/1 -> Gain/1, Math Function/1, Product1/1, Product3/2, Integrator1/1  "omega"
  Integrator1/1 -> Sine/1  "theta"
  Gain/1 -> "Propeller model "/1(rpm), rpm/1  "rpm"
  J/1 -> Divide/2  "J"
  d/1 -> Product/2  "d"
  Math Function/1 -> Product/1
  Df/1 -> Product1/2  "Df"
  Tf/1 -> Sum/4  "Tf"
  Ke/1 -> Product3/1, Product2/2  "Ke"
  Product2/1 -> Display1/1, Sum/1
  Divide1/1 -> Product2/1, MATLAB Function/1(u)  "current"
  V/1 -> MATLAB Function1/1(u)  "V"
  Product3/1 -> Sum1/2
  MATLAB Function/1(y) -> current/1  "current"
  MATLAB Function1/1(y) -> Sum1/1  "vb"
  Sum1/1 -> Divide1/1
  R/1 -> Divide1/2
  "Propeller model "/2(thrust) -> thrust/1
  "Propeller model "/1(torque) -> torque/1
  Product1/1 -> Sum/3
  Product/1 -> Display2/1, Sum/2
  Sum/1 -> Display/1, Divide/1

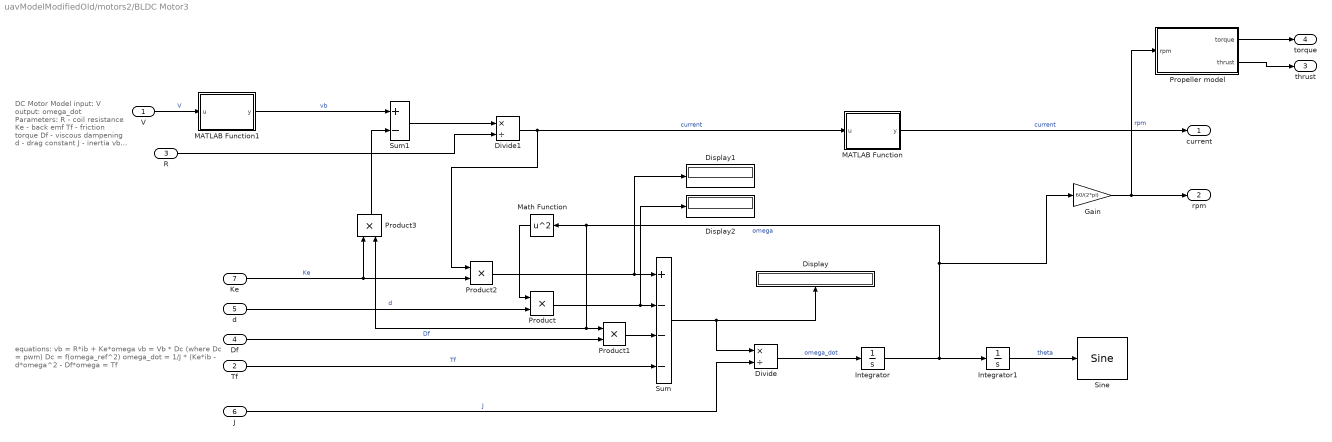
== system uavModelModifiedOld/motors2/BLDC Motor3 ==
  note: DC Motor Model
      |
      | input:
      | V
      |
      | output:
      | omega_dot
      |
      | Parameters:
      | R   - coil resistance
      | Ke - back emf
      | Tf  - friction torque
      | Df  - viscous dampening
      | d   - drag constant
      | J   - inertia
      |
      |
      | vb - average battery voltage
      | ib  - average battery current
  note: equations:
      |
      | vb = R*ib + Ke*omega
      | vb = Vb * Dc  (where Dc = pwm)
      | Dc = f(omega_ref^2)
      |
      | omega_dot = 1/J * (Ke*ib - d*omega^2 - Df*omega = Tf
  V : Inport
  Tf : Inport  Port=2
  R : Inport  Port=3
  Df : Inport  Port=4
  d : Inport  Port=5
  J : Inport  Port=6
  Ke : Inport  Port=7
  Display : Display
  Display1 : Display
  Display2 : Display
  Divide : Product  Inputs=*/
  Divide1 : Product  Inputs=*/
  Gain : Gain  Gain=60/(2*pi)
  Integrator : Integrator
  Integrator1 : Integrator
  MATLAB Function : MATLAB Function  TreatAsAtomicUnit=on
  MATLAB Function1 : MATLAB Function  TreatAsAtomicUnit=on
  Math Function : Math  Operator=square  SaturateOnIntegerOverflow=on
  Product{,1..3} (4 alike) : Product
  "Propeller model " : MATLAB Function  TreatAsAtomicUnit=on
  Sine : simulink/Lookup Tables/Sine  Formula=sin(2*pi*u)  NumDataPoints=180  OutputWordLength=16  InternalRulePriority=Speed
      settings: SourceProductName=Simulink
  Sum : Sum  Inputs=+---
  Sum1 : Sum  Inputs=+-
  current : Outport
  rpm : Outport  Port=2
  thrust : Outport  Port=3
  torque : Outport  Port=4
  wires:
  Divide/1 -> Integrator/1  "omega_dot"
  Integrator/1 -> Gain/1, Math Function/1, Product1/1, Product3/2, Integrator1/1  "omega"
  Integrator1/1 -> Sine/1  "theta"
  Gain/1 -> "Propeller model "/1(rpm), rpm/1  "rpm"
  J/1 -> Divide/2  "J"
  d/1 -> Product/2  "d"
  Math Function/1 -> Product/1
  Df/1 -> Product1/2  "Df"
  Tf/1 -> Sum/4  "Tf"
  Ke/1 -> Product3/1, Product2/2  "Ke"
  Product2/1 -> Display1/1, Sum/1
  Divide1/1 -> Product2/1, MATLAB Function/1(u)  "current"
  V/1 -> MATLAB Function1/1(u)  "V"
  Product3/1 -> Sum1/2
  MATLAB Function/1(y) -> current/1  "current"
  MATLAB Function1/1(y) -> Sum1/1  "vb"
  Sum1/1 -> Divide1/1
  R/1 -> Divide1/2
  "Propeller model "/2(thrust) -> thrust/1
  "Propeller model "/1(torque) -> torque/1
  Product1/1 -> Sum/3
  Product/1 -> Display2/1, Sum/2
  Sum/1 -> Display/1, Divide/1

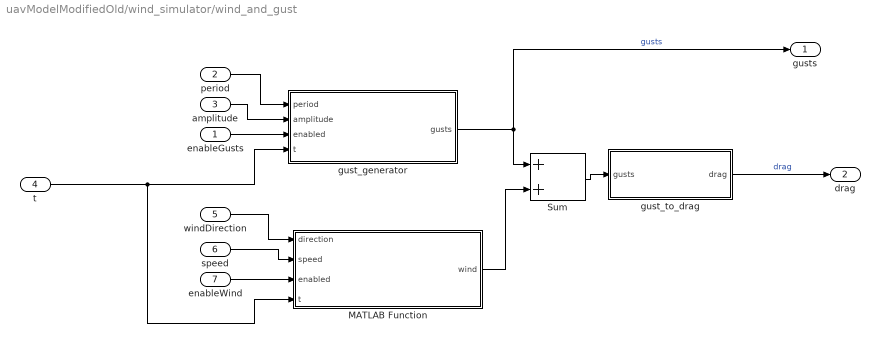
== system uavModelModifiedOld/wind_simulator/wind_and_gust ==
  enableGusts : Inport
  period : Inport  Port=2
  amplitude : Inport  Port=3
  t : Inport  Port=4
  windDirection : Inport  Port=5
  speed : Inport  Port=6
  enableWind : Inport  Port=7
  MATLAB Function : MATLAB Function  TreatAsAtomicUnit=on
  Sum : Sum
  gust_generator : MATLAB Function  TreatAsAtomicUnit=on
  gust_to_drag : MATLAB Function  TreatAsAtomicUnit=on
  gusts : Outport
  drag : Outport  Port=2
  wires:
  period/1 -> gust_generator/1(period)
  gust_generator/1(gusts) -> Sum/1, gusts/1  "gusts"
  enableGusts/1 -> gust_generator/3(enabled)
  gust_to_drag/1(drag) -> drag/1  "drag"
  t/1 -> gust_generator/4(t), MATLAB Function/4(t)
  amplitude/1 -> gust_generator/2(amplitude)
  Sum/1 -> gust_to_drag/1(gusts)
  MATLAB Function/1(wind) -> Sum/2
  windDirection/1 -> MATLAB Function/1(direction)
  speed/1 -> MATLAB Function/2(speed)
  enableWind/1 -> MATLAB Function/3(enabled)

== system uavModelModifiedOld/Motors1/motorRotor1/Electrical part ==
  ESC voltage : Inport
  w angular speed : Inport  Port=2
  1/R : Gain  Gain=1/Motor.Req
  Ke (Torque constant)1 : Gain  Gain=Motor.Ke_eq
  Kt (Torque constant) Kt=Ke for an ideal square wave motor : Gain  Gain=Motor.Ke_eq
  Sum : Sum  Inputs=|+-
  Electrical Torque : Outport
  current : Outport  Port=2
  wires:
  1/R/1 -> current/1, Kt (Torque constant) Kt=Ke for an ideal square wave motor/1  "current i"
  Sum/1 -> 1/R/1
  Kt (Torque constant) Kt=Ke for an ideal square wave motor/1 -> Electrical Torque/1
  Ke (Torque constant)1/1 -> Sum/2
  ESC voltage/1 -> Sum/1
  w angular speed/1 -> Ke (Torque constant)1/1

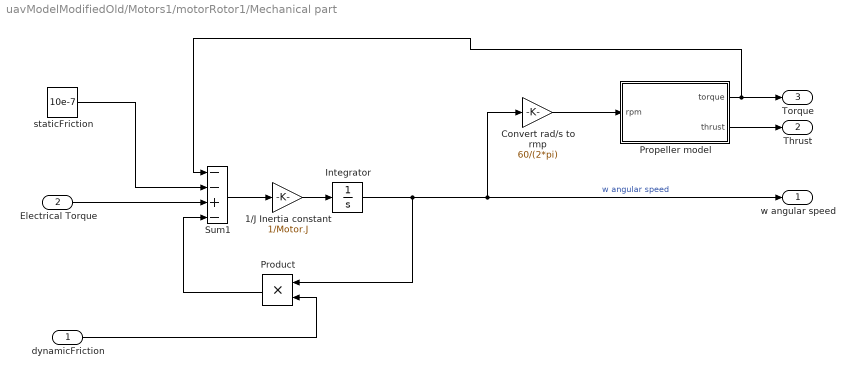
== system uavModelModifiedOld/Motors1/motorRotor1/Mechanical part ==
  dynamicFriction : Inport
  Electrical Torque : Inport  Port=2
  1/J Inertia constant : Gain  Gain=1/Motor.J
  Convert rad/s to rmp : Gain  Gain=60/(2*pi)
  Integrator : Integrator
  Product : Product
  "Propeller model " : MATLAB Function  TreatAsAtomicUnit=on
  Sum1 : Sum  Inputs=--+-
  staticFriction : Constant  Value=10e-7
  w angular speed : Outport
  Thrust : Outport  Port=2
  Torque : Outport  Port=3
  wires:
  "Propeller model "/1(torque) -> Sum1/1, Torque/1
  1/J Inertia constant/1 -> Integrator/1
  dynamicFriction/1 -> Product/2
  Product/1 -> Sum1/4
  Integrator/1 -> Product/1, w angular speed/1, Convert rad/s to rmp/1  "w angular speed"
  Sum1/1 -> 1/J Inertia constant/1
  Electrical Torque/1 -> Sum1/3
  Convert rad/s to rmp/1 -> "Propeller model "/1(rpm)
  "Propeller model "/2(thrust) -> Thrust/1
  staticFriction/1 -> Sum1/2

== system uavModelModifiedOld/Motors1/motorRotor2/Electrical part ==
  ESC voltage : Inport
  w angular speed : Inport  Port=2
  1/R : Gain  Gain=1/Motor.Req
  Ke (Torque constant)1 : Gain  Gain=Motor.Ke_eq
  Kt (Torque constant) Kt=Ke for an ideal square wave motor : Gain  Gain=Motor.Ke_eq
  Sum : Sum  Inputs=|+-
  Electrical Torque : Outport
  current : Outport  Port=2
  wires:
  1/R/1 -> current/1, Kt (Torque constant) Kt=Ke for an ideal square wave motor/1  "current i"
  Sum/1 -> 1/R/1
  Kt (Torque constant) Kt=Ke for an ideal square wave motor/1 -> Electrical Torque/1
  Ke (Torque constant)1/1 -> Sum/2
  ESC voltage/1 -> Sum/1
  w angular speed/1 -> Ke (Torque constant)1/1

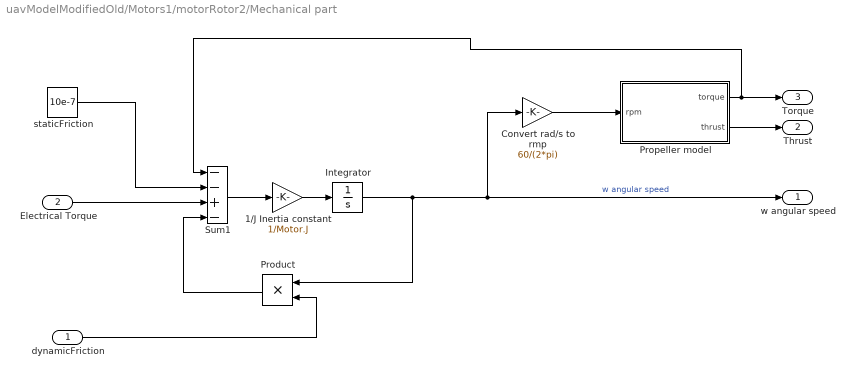
== system uavModelModifiedOld/Motors1/motorRotor2/Mechanical part ==
  dynamicFriction : Inport
  Electrical Torque : Inport  Port=2
  1/J Inertia constant : Gain  Gain=1/Motor.J
  Convert rad/s to rmp : Gain  Gain=60/(2*pi)
  Integrator : Integrator
  Product : Product
  "Propeller model " : MATLAB Function  TreatAsAtomicUnit=on
  Sum1 : Sum  Inputs=--+-
  staticFriction : Constant  Value=10e-7
  w angular speed : Outport
  Thrust : Outport  Port=2
  Torque : Outport  Port=3
  wires:
  "Propeller model "/1(torque) -> Sum1/1, Torque/1
  1/J Inertia constant/1 -> Integrator/1
  dynamicFriction/1 -> Product/2
  Product/1 -> Sum1/4
  Integrator/1 -> Product/1, w angular speed/1, Convert rad/s to rmp/1  "w angular speed"
  Sum1/1 -> 1/J Inertia constant/1
  Electrical Torque/1 -> Sum1/3
  Convert rad/s to rmp/1 -> "Propeller model "/1(rpm)
  "Propeller model "/2(thrust) -> Thrust/1
  staticFriction/1 -> Sum1/2

== system uavModelModifiedOld/Motors1/motorRotor3/Electrical part ==
  ESC voltage : Inport
  w angular speed : Inport  Port=2
  1/R : Gain  Gain=1/Motor.Req
  Ke (Torque constant)1 : Gain  Gain=Motor.Ke_eq
  Kt (Torque constant) Kt=Ke for an ideal square wave motor : Gain  Gain=Motor.Ke_eq
  Sum : Sum  Inputs=|+-
  Electrical Torque : Outport
  current : Outport  Port=2
  wires:
  1/R/1 -> current/1, Kt (Torque constant) Kt=Ke for an ideal square wave motor/1  "current i"
  Sum/1 -> 1/R/1
  Kt (Torque constant) Kt=Ke for an ideal square wave motor/1 -> Electrical Torque/1
  Ke (Torque constant)1/1 -> Sum/2
  ESC voltage/1 -> Sum/1
  w angular speed/1 -> Ke (Torque constant)1/1

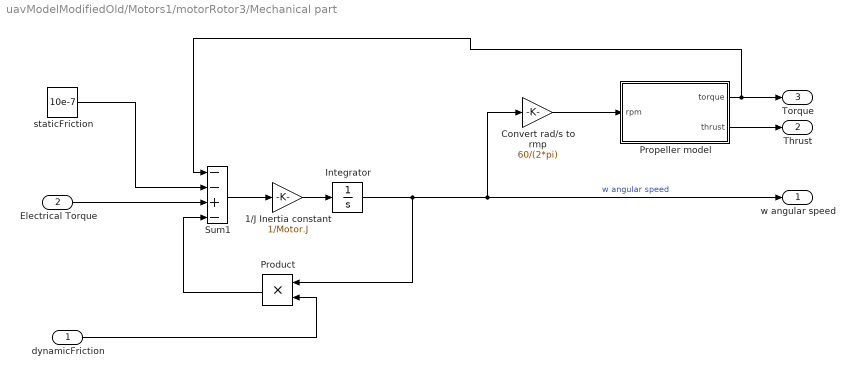
== system uavModelModifiedOld/Motors1/motorRotor3/Mechanical part ==
  dynamicFriction : Inport
  Electrical Torque : Inport  Port=2
  1/J Inertia constant : Gain  Gain=1/Motor.J
  Convert rad/s to rmp : Gain  Gain=60/(2*pi)
  Integrator : Integrator
  Product : Product
  "Propeller model " : MATLAB Function  TreatAsAtomicUnit=on
  Sum1 : Sum  Inputs=--+-
  staticFriction : Constant  Value=10e-7
  w angular speed : Outport
  Thrust : Outport  Port=2
  Torque : Outport  Port=3
  wires:
  "Propeller model "/1(torque) -> Sum1/1, Torque/1
  1/J Inertia constant/1 -> Integrator/1
  dynamicFriction/1 -> Product/2
  Product/1 -> Sum1/4
  Integrator/1 -> Product/1, w angular speed/1, Convert rad/s to rmp/1  "w angular speed"
  Sum1/1 -> 1/J Inertia constant/1
  Electrical Torque/1 -> Sum1/3
  Convert rad/s to rmp/1 -> "Propeller model "/1(rpm)
  "Propeller model "/2(thrust) -> Thrust/1
  staticFriction/1 -> Sum1/2

== system uavModelModifiedOld/Motors1/motorRotor4/Electrical part ==
  ESC voltage : Inport
  w angular speed : Inport  Port=2
  1/R : Gain  Gain=1/Motor.Req
  Ke (Torque constant)1 : Gain  Gain=Motor.Ke_eq
  Kt (Torque constant) Kt=Ke for an ideal square wave motor : Gain  Gain=Motor.Ke_eq
  Sum : Sum  Inputs=|+-
  Electrical Torque : Outport
  current : Outport  Port=2
  wires:
  1/R/1 -> current/1, Kt (Torque constant) Kt=Ke for an ideal square wave motor/1  "current i"
  Sum/1 -> 1/R/1
  Kt (Torque constant) Kt=Ke for an ideal square wave motor/1 -> Electrical Torque/1
  Ke (Torque constant)1/1 -> Sum/2
  ESC voltage/1 -> Sum/1
  w angular speed/1 -> Ke (Torque constant)1/1

== system uavModelModifiedOld/Motors1/motorRotor4/Mechanical part ==
  dynamicFriction : Inport
  Electrical Torque : Inport  Port=2
  1/J Inertia constant : Gain  Gain=1/Motor.J
  Convert rad/s to rmp : Gain  Gain=60/(2*pi)
  Integrator : Integrator
  Product : Product
  "Propeller model " : MATLAB Function  TreatAsAtomicUnit=on
  Sum1 : Sum  Inputs=--+-
  staticFriction : Constant  Value=10e-7
  w angular speed : Outport
  Thrust : Outport  Port=2
  Torque : Outport  Port=3
  wires:
  "Propeller model "/1(torque) -> Sum1/1, Torque/1
  1/J Inertia constant/1 -> Integrator/1
  dynamicFriction/1 -> Product/2
  Product/1 -> Sum1/4
  Integrator/1 -> Product/1, w angular speed/1, Convert rad/s to rmp/1  "w angular speed"
  Sum1/1 -> 1/J Inertia constant/1
  Electrical Torque/1 -> Sum1/3
  Convert rad/s to rmp/1 -> "Propeller model "/1(rpm)
  "Propeller model "/2(thrust) -> Thrust/1
  staticFriction/1 -> Sum1/2

== matlab function uavModelModifiedOld/angular_acceleration_calculation ==
  data: thrust input; torque input; angular_acceleration output
function angular_acceleration = calc_angular_acceleration(thrust, torque)
%
% inputs: torque vector
%         thrust vector
%
% output: rotational acceleration (of drone)
%

% moments about each axis (x,y,z) i.e. (pitch, roll, yaw)
moments = [0 0 0];

% rotational acceleration about each axis
angular_acceleration = [0 0 0];

% moments of inertia empirically derived from sample data
moments_I = [.003, .003, .007];

% pitch
% motor pair A * 1/2 rigid body length - motor pair B * rigid body length
moments(1) = (thrust(3) + thrust(4))*.237/2 - (thrust(1)+thrust(2))*.237/2;
% roll
% motor pair A * 1/2 rigid body length - motor pair B * rigid body length
moments(2) = (thrust(3) + thrust(2))*.237/2 - (thrust(1)+thrust(4))*.237/2;
%yaw
% motor pair A - motor pair B
moments(3) = (torque(4) + torque(2)) - (torque(1)  + torque(3));

for i=1:3
    angular_acceleration(i) = moments(i) / moments_I(i);
end

== matlab function uavModelModifiedOld/original_motor_model ==
  data: voltage input; thrust output; rpm output; torque output; current output; Tf input
function [thrust, rpm, torque, current] = calc_thrust_torque_current(voltage, Tf)
%
% input: voltage
%
% output: motor torque, 
%         propeller thrust 
%         battery current
%

% rpm constant
KV = 1400;
% per motor
rpm = [0 0 0 0]; 
thrust = [0 0 0 0];
torque = [0 0 0 0];
current = [0 0 0 0];


for i=1:4
    % empirically derived equation given sample data
    rpm(i) = -2.6931*voltage(i)^3 + KV*voltage(i);
    %coefficient of thrust, empirically derived
    coef_t = 2*(10^-15)*rpm(i)^3 - 4*(10^-11)*rpm(i)^2 + 3*(10^-7)*rpm(i) + .1013;
    %thrust = coef_t * density of air * velocity^2 * propeller diameter (m) ^4
    thrust(i) = coef_t*1.225*(rpm(i)/60)^2*.2^4;
    % empirically derived
    torque(i) = 4*(10^-14)*rpm(i)^3 +  8*(10^-12)*rpm(i)^2 + 3*(10^-6)*rpm(i);
    % current = rpm constant * torque
    current(i) = KV*torque(i);
end

== matlab function uavModelModifiedOld/linear_acceleration_calculation ==
  data: thrust input; linear_acceleration output; disturbances input; theta input; linear_velocity input
function linear_acceleration = calc_linear_acceleration(thrust, disturbances, theta, linear_velocity)
%
% inputs: thrust vector (m1, m2, m3, m4)
%         disturbances vector (x,y,z)
%         theta vector (x,y,z)
%         linear velocity vector (x,y,z)
%
% output: linear acceleration vector (x,y,z)
%

m = .743; % mass of drone
g = 9.81; % acceleration due to gravity
rho = 1.225; % density of air at sea level
coef_d = 1.0; % coefficient of drag for the drone

% cross sectional areas of drone in x,y,z planes
areas = [.0197, .0197, .0512];

linear_acceleration = [0 0 0];
force = [0 0 0];
xyz_thrust = [0;0;0];
drag = [0 0 0];

% trigonometric functions for calculating pitch,roll,yaw (x,y,z) thrust 
xyz_thrust(1,1) = sin(theta(2))*cos(theta(1))*sum(thrust);
xyz_thrust(2,1) = sin(theta(1))*cos(theta(2))*sum(thrust);
xyz_thrust(3,1) = cos(theta(1))*cos(theta(2))*sum(thrust);

% angular position and magnitude on the pitch-roll (x,y) plane
angular_pos =-atan2(xyz_thrust(1), xyz_thrust(2));
angular_mag = sqrt(xyz_thrust(1)^2 + xyz_thrust(2)^2);

% if the drone is pointed upwards, x and y thrust uses + theta(3) (z)
if(xyz_thrust(3) >= 0)
    xyz_thrust(1) = angular_mag * sin(angular_pos + theta(3));
    xyz_thrust(2) = angular_mag * cos(angular_pos + theta(3));
else
    xyz_thrust(1) = angular_mag * sin(angular_pos - theta(3));
    xyz_thrust(2) = angular_mag * cos(angular_pos - theta(3));  
end

% calculate drage and force in x,y,z 
for i=1:3
    drag(i) = .5*rho*linear_velocity(i)^2* areas(i)*coef_d;
    % if the drone is going backward (w.r.t its local coordinate system)
    if (linear_velocity(i) < 0)
        force(i) = xyz_thrust(i) - disturbances(i) + drag(i);
    else
        force(i) = xyz_thrust(i) - disturbances(i) - drag(i);
    end
    % account for gravity in the z direction
    if(i == 3)
        force(i) = force(i) - m*g;
    end
end

%f=ma to calculate final acceleration
for i=1:3
    linear_acceleration(i) = force(i)/m;
end

== matlab function uavModelModifiedOld/wind_simulator/wind_and_gust/gust_to_drag ==
  data: gusts input; drag output
function drag = gust_to_drag(gusts)
%
% creates drag from wind gusts
%
% input: gusts (x,y,z)
%
% output: drag (x,y,z)
%

areas = [.0197 .0197 .0197*2*1.3];
drag = [0 0 0];
rho = 1.225;
coef_d = 1.0;

for i=1:3
    drag(i) = .5*rho*gusts(i)^2*areas(i)*coef_d;
    if(gusts(i)>0)
        drag(i) = drag(i) * -1;
    end   
end

== matlab function uavModelModifiedOld/control_mixer ==
  data: throttle input; pitch input; roll input; yaw input; Vbatt input; motor_voltage output
function motor_voltage = control_mixer(throttle, pitch, roll, yaw, Vbatt)
%
% outputs voltage per motor given control inputs
%
% inputs: throttle (double)
%         pitch (double)
%         roll (double)
%         yaw (double)
%
% output: voltage vector (m1 m2 m3 m4)
%

%battery voltage
BATT_V = Vbatt;

bias = 0.0;

% pitch, roll, and yaw inputs, /2 due to drone symmetry w.r.t 4 motors
xyz_input = (pitch + roll + yaw )/2;

% difference between max throttle (100%) and current throttle
throttle_diff = 100 - throttle;

% throttle is most important, so excess is for pitch/roll/yaw
if(xyz_input > throttle_diff)
    bias = xyz_input - throttle_diff; 
end

% if the input is greater than throttle, set the bias to input-throttle
if(xyz_input > (throttle))
    if(bias < (xyz_input - throttle))
        bias = xyz_input - throttle;
    end
end

% set the bias for each motor and attitude value (pitch,roll,yaw)
bias = 2*bias/3;

%update the input commands 
if (bias ~= 0.0)
    pitch = pitch - bias;
    roll = roll - bias;
    yaw = yaw - bias;
end

motor_voltage = [(throttle - pitch/2 - roll/2 - yaw/2)*BATT_V/100
                 (throttle - pitch/2 + roll/2 + yaw/2)*BATT_V/100
                 (throttle + pitch/2 + roll/2 - yaw/2)*BATT_V/100
                 (throttle + pitch/2 - roll/2 + yaw/2)*BATT_V/100];

== matlab function uavModelModifiedOld/Motors1/motorRotor1/Mechanical part/Propeller model  ==
  data: torque output; rpm input; thrust output
function [torque,thrust] = fcn(rpm)
% angular_velocity in rpm

%coefficient of thrust, empirically derived
coef_t = 2*(10^-15)*rpm^3 - 4*(10^-11)*rpm^2 + 3*(10^-7)*rpm + .1013;
%thrust = coef_t * density of air * velocity^2 * propeller diameter (m) ^4
thrust = coef_t*1.225*(rpm/60)^2*.2^4;
% empirically derived
torque = 4*(10^-14)*rpm^3 +  8*(10^-12)*rpm^2 + 3*(10^-6)*rpm;
end

== matlab function uavModelModifiedOld/Motors1/motorRotor2/Mechanical part/Propeller model  ==
  data: torque output; rpm input; thrust output
function [torque,thrust] = fcn(rpm)
% angular_velocity in rpm

%coefficient of thrust, empirically derived
coef_t = 2*(10^-15)*rpm^3 - 4*(10^-11)*rpm^2 + 3*(10^-7)*rpm + .1013;
%thrust = coef_t * density of air * velocity^2 * propeller diameter (m) ^4
thrust = coef_t*1.225*(rpm/60)^2*.2^4;
% empirically derived
torque = 4*(10^-14)*rpm^3 +  8*(10^-12)*rpm^2 + 3*(10^-6)*rpm;
end

== matlab function uavModelModifiedOld/Motors1/motorRotor3/Mechanical part/Propeller model  ==
  data: torque output; rpm input; thrust output
function [torque,thrust] = fcn(rpm)
% angular_velocity in rpm

%coefficient of thrust, empirically derived
coef_t = 2*(10^-15)*rpm^3 - 4*(10^-11)*rpm^2 + 3*(10^-7)*rpm + .1013;
%thrust = coef_t * density of air * velocity^2 * propeller diameter (m) ^4
thrust = coef_t*1.225*(rpm/60)^2*.2^4;
% empirically derived
torque = 4*(10^-14)*rpm^3 +  8*(10^-12)*rpm^2 + 3*(10^-6)*rpm;
end

== matlab function uavModelModifiedOld/friction_fault_generator ==
  settings: updateMethod=DISCRETE
  data: motor_select input; onset input; enabled input; t input; Tf output
function Tf = friction_fault_generator(motor_select, onset, enabled, t)

Tf = [1e-8,1e-8,1e-8,1e-8];

if enabled == 1
    Tf(motor_select) = onset * t;
end

== matlab function uavModelModifiedOld/wind_simulator/wind_and_gust/gust_generator ==
  settings: updateMethod=DISCRETE
  data: period input; amplitude input; enabled input; gusts output; t input
function gusts = gust_generator(period, amplitude, enabled, t)

gusts = [0,0,0];
idx = 0;

if enabled == 1
    if mod(t,period) == 0
        if rand > .8
            select = rand;
            if select < .3333
                idx = 1;
            elseif select > .6666
                idx = 3;
            else
                idx = 2;
            end % create a gust
            gusts(idx) = normrnd(0, amplitude);
        end
    end
end

== matlab function uavModelModifiedOld/motors2/BLDC Motor/MATLAB Function ==
  data: u input; y output
function y = Dc(u)

y = 1*u;

== matlab function uavModelModifiedOld/motors2/BLDC Motor/MATLAB Function1 ==
  data: u input; y output
function y = Dc(u)

y = 1*u;

== matlab function uavModelModifiedOld/motors2/BLDC Motor/Propeller model  ==
  data: torque output; rpm input; thrust output
function [torque,thrust] = fcn(rpm)
% angular_velocity in rpm

%coefficient of thrust, empirically derived
coef_t = 2*(10^-15)*rpm^3 - 4*(10^-11)*rpm^2 + 3*(10^-7)*rpm + .1013;
%thrust = coef_t * density of air * velocity^2 * propeller diameter (m) ^4
thrust = coef_t*1.225*(rpm/60)^2*.2^4;
% empirically derived
torque = 4*(10^-14)*rpm^3 +  8*(10^-12)*rpm^2 + 3*(10^-6)*rpm;
end

== matlab function uavModelModifiedOld/motors2/BLDC Motor1/MATLAB Function ==
  data: u input; y output
function y = Dc(u)

y = 1*u;

== matlab function uavModelModifiedOld/Motors1/motorRotor4/Mechanical part/Propeller model  ==
  data: torque output; rpm input; thrust output
function [torque,thrust] = fcn(rpm)
% angular_velocity in rpm

%coefficient of thrust, empirically derived
coef_t = 2*(10^-15)*rpm^3 - 4*(10^-11)*rpm^2 + 3*(10^-7)*rpm + .1013;
%thrust = coef_t * density of air * velocity^2 * propeller diameter (m) ^4
thrust = coef_t*1.225*(rpm/60)^2*.2^4;
% empirically derived
torque = 4*(10^-14)*rpm^3 +  8*(10^-12)*rpm^2 + 3*(10^-6)*rpm;
end

== matlab function uavModelModifiedOld/motors2/BLDC Motor1/MATLAB Function1 ==
  data: u input; y output
function y = Dc(u)

y = 1*u;

== matlab function uavModelModifiedOld/motors2/BLDC Motor1/Propeller model  ==
  data: torque output; rpm input; thrust output
function [torque,thrust] = fcn(rpm)
% angular_velocity in rpm

%coefficient of thrust, empirically derived
coef_t = 2*(10^-15)*rpm^3 - 4*(10^-11)*rpm^2 + 3*(10^-7)*rpm + .1013;
%thrust = coef_t * density of air * velocity^2 * propeller diameter (m) ^4
thrust = coef_t*1.225*(rpm/60)^2*.2^4;
% empirically derived
torque = 4*(10^-14)*rpm^3 +  8*(10^-12)*rpm^2 + 3*(10^-6)*rpm;
end

== matlab function uavModelModifiedOld/motors2/BLDC Motor2/MATLAB Function ==
  data: u input; y output
function y = Dc(u)

y = 1*u;

== matlab function uavModelModifiedOld/motors2/BLDC Motor2/MATLAB Function1 ==
  data: u input; y output
function y = Dc(u)

y = 1*u;
